simulink model "VoltageDivider_sim_2020"  (R2020b)
settings: Solver=ode4  StartTime=0.0  StopTime=2  FixedStep=0.05  RelTol=1e-3
settings Model: Creator=005274  LastModifiedBy=005274

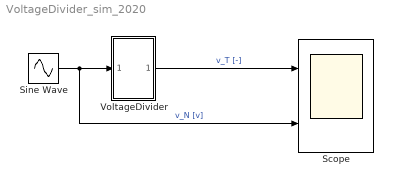
== system VoltageDivider_sim_2020 ==
  Scope : Scope  NumInputPorts=2
  Sine Wave : Sin  Amplitude=5  Bias=5  Frequency=2*pi  SampleTime=0
  VoltageDivider : Subsystem  mask{alpha=0.5}
  wires:
  VoltageDivider/1(Out1) -> Scope/1  "v_T [-]"
  Sine Wave/1 -> Scope/2, VoltageDivider/1(In1)  "v_N [v]"

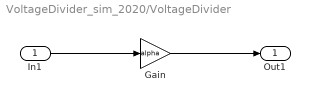
== system VoltageDivider_sim_2020/VoltageDivider ==
  In1 : Inport
  Gain : Gain  Gain=alpha
  Out1 : Outport
  wires:
  In1/1 -> Gain/1
  Gain/1 -> Out1/1
